simulink model "W03_4_teleop"  (R2024b)
settings: Solver=FixedStepDiscrete  StartTime=0.0  StopTime=T_end_teleop  FixedStep=Ts  RelTol=1e-3
values from neighbouring files (symbols this model uses):
  animate = 1    [W03_setup.m]
  teleop_thrust = 200    [W03_setup.m]
  Ts = 0.05    [W03_setup.m]
libraries: ros2lib x5
settings Model: Creator=admin  LastModifiedBy=admin

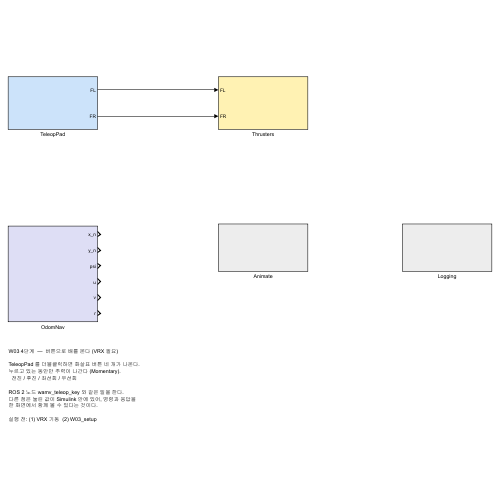
[thumbnail: Simulink's stored preview of the top-level diagram]
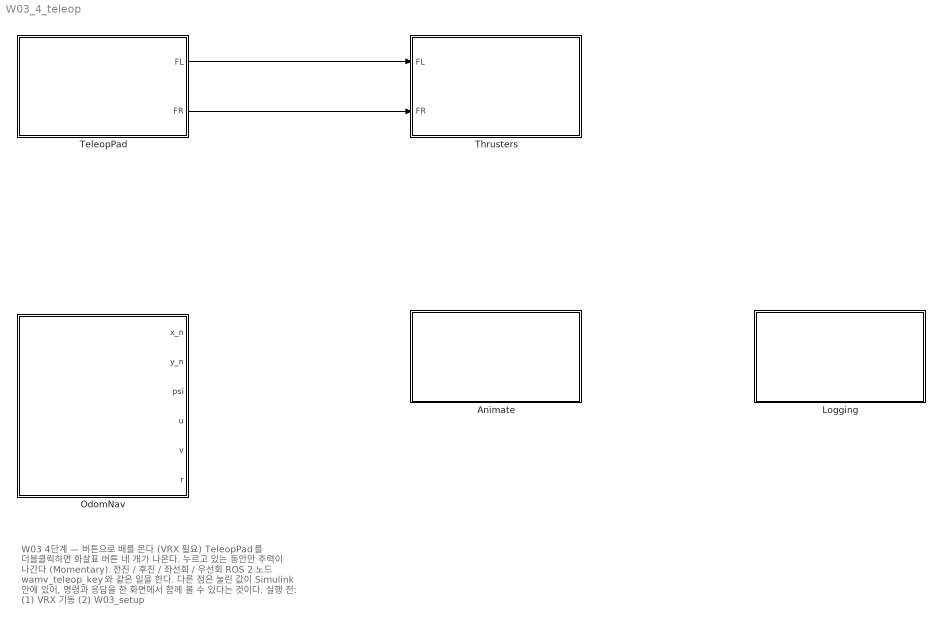
== system W03_4_teleop ==
  note: W03 4단계  —  버튼으로 배를 몬다 (VRX 필요)
      |
      | TeleopPad 를 더블클릭하면 화살표 버튼 네 개가 나온다.
      | 누르고 있는 동안만 추력이 나간다 (Momentary).
      |   전진 / 후진 / 좌선회 / 우선회
      |
      | ROS 2 노드 wamv_teleop_key 와 같은 일을 한다.
      | 다른 점은 눌린 값이 Simulink 안에 있어, 명령과 응답을
      | 한 화면에서 함께 볼 수 있다는 것이다.
      |
      | 실행 전: (1) VRX 기동  (2) W03_setup
  Animate : Subsystem
  Logging : Subsystem
  OdomNav : Subsystem
  TeleopPad : Subsystem
  Thrusters : Subsystem
  wires:
  TeleopPad/1(FL) -> Thrusters/1(FL)
  TeleopPad/2(FR) -> Thrusters/2(FR)

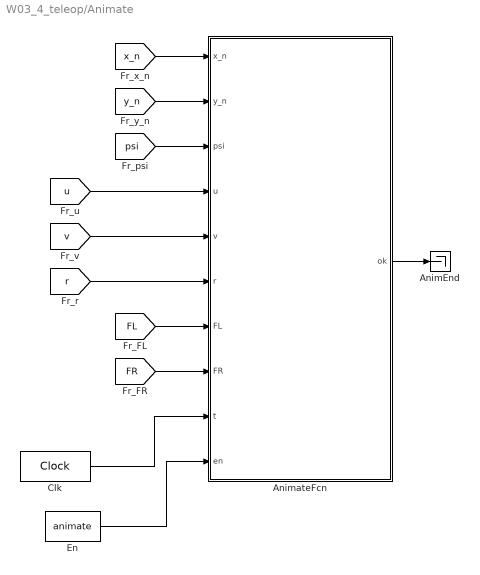
== system W03_4_teleop/Animate ==
  AnimEnd : Terminator
  AnimateFcn : MATLAB Function  TreatAsAtomicUnit=on
  Clk : DigitalClock  SampleTime=Ts
  En : Constant  Value=animate
  wires:
  [r] -> AnimateFcn/6(r)
  [u] -> AnimateFcn/4(u)
  [v] -> AnimateFcn/5(v)
  Clk/1 -> AnimateFcn/9(t)
  En/1 -> AnimateFcn/10(en)
  AnimateFcn/1(ok) -> AnimEnd/1
  [FL] -> AnimateFcn/7(FL)
  [FR] -> AnimateFcn/8(FR)
  [psi] -> AnimateFcn/3(psi)
  [y_n] -> AnimateFcn/2(y_n)
  [x_n] -> AnimateFcn/1(x_n)

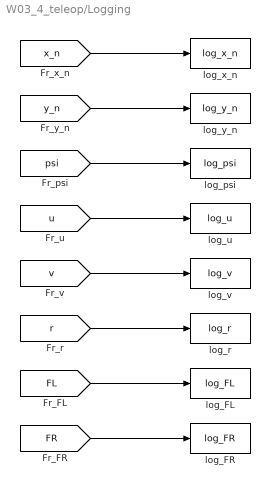
== system W03_4_teleop/Logging ==
  log_FL : ToWorkspace  VariableName=log_FL  SaveFormat=Timeseries  SampleTime=Ts
  log_FR : ToWorkspace  VariableName=log_FR  SaveFormat=Timeseries  SampleTime=Ts
  log_psi : ToWorkspace  VariableName=log_psi  SaveFormat=Timeseries  SampleTime=Ts
  log_r : ToWorkspace  VariableName=log_r  SaveFormat=Timeseries  SampleTime=Ts
  log_u : ToWorkspace  VariableName=log_u  SaveFormat=Timeseries  SampleTime=Ts
  log_v : ToWorkspace  VariableName=log_v  SaveFormat=Timeseries  SampleTime=Ts
  log_x_n : ToWorkspace  VariableName=log_x_n  SaveFormat=Timeseries  SampleTime=Ts
  log_y_n : ToWorkspace  VariableName=log_y_n  SaveFormat=Timeseries  SampleTime=Ts
  wires:
  [x_n] -> log_x_n/1
  [y_n] -> log_y_n/1
  [psi] -> log_psi/1
  [u] -> log_u/1
  [v] -> log_v/1
  [r] -> log_r/1
  [FL] -> log_FL/1
  [FR] -> log_FR/1

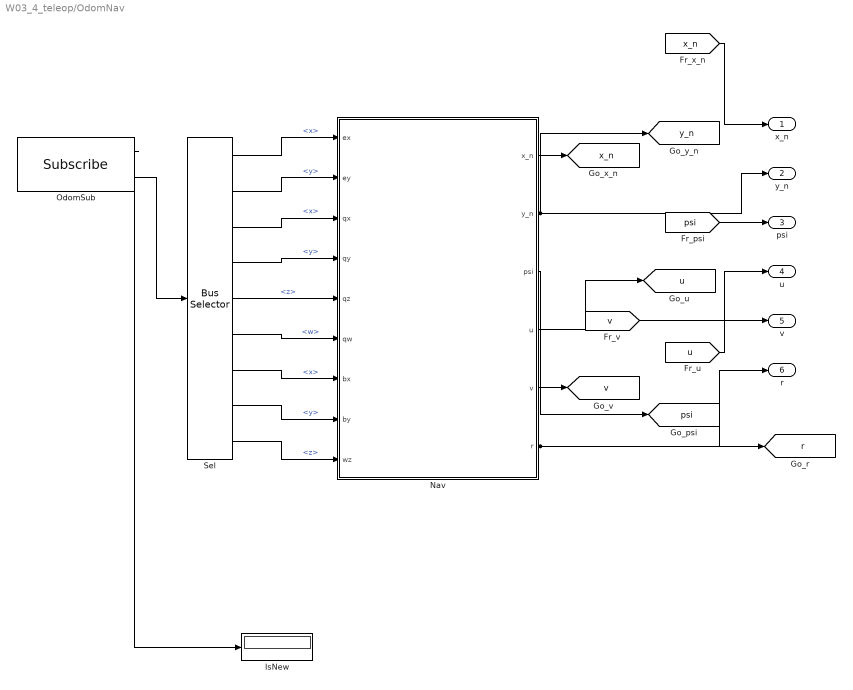
== system W03_4_teleop/OdomNav ==
  IsNew : Display
  Nav : MATLAB Function  TreatAsAtomicUnit=on
  OdomSub : ros2lib/Subscribe  topicSource=Specify your own  topic=/wamv/sensors/position/ground_truth_odometry  messageType=nav_msgs/Odometry  sampleTime=Ts  QOSHistory=Keep last  QOSDepth=1  QOSReliability=Reliable  QOSDurability=Volatile  QOSDeadline=Inf  QOSLifespan=Inf  QOSLiveliness=Automatic  QOSLeaseDuration=Inf  QOSAvoidROSNamespaceConventions=off
  Sel : BusSelector  OutputSignals=pose.pose.position.x,pose.pose.position.y,pose.pose.orientation.x,pose.pose.orientation.y,pose.pose.orientation.z,pose.pose.orientation.w,twist.twist.linear.x,twist.twist.linear.y,twist.twist.angular.z
  x_n : Outport
  y_n : Outport  Port=2
  psi : Outport  Port=3
  u : Outport  Port=4
  v : Outport  Port=5
  r : Outport  Port=6
  tag scope: psi=global, r=global, u=global, v=global, x_n=global, y_n=global
  wires:
  OdomSub/2 -> Sel/1
  Sel/1 -> Nav/1(ex)  "<x>"
  Sel/2 -> Nav/2(ey)  "<y>"
  Sel/3 -> Nav/3(qx)  "<x>"
  Sel/4 -> Nav/4(qy)  "<y>"
  Sel/5 -> Nav/5(qz)  "<z>"
  Sel/6 -> Nav/6(qw)  "<w>"
  Sel/7 -> Nav/7(bx)  "<x>"
  Sel/8 -> Nav/8(by)  "<y>"
  Sel/9 -> Nav/9(wz)  "<z>"
  Nav/2(y_n) -> y_n/1, [y_n]
  Nav/4(u) -> [u]
  OdomSub/1 -> IsNew/1
  Nav/5(v) -> [v]
  Nav/1(x_n) -> [x_n]
  [psi] -> psi/1
  [v] -> v/1
  Nav/6(r) -> [r], r/1
  Nav/3(psi) -> [psi]
  [u] -> u/1
  [x_n] -> x_n/1

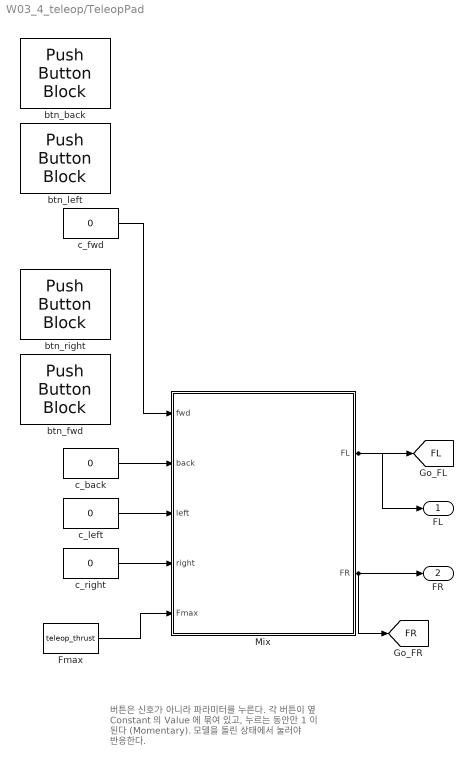
== system W03_4_teleop/TeleopPad ==
  note: 버튼은 신호가 아니라 파라미터를 누른다.
      | 각 버튼이 옆 Constant 의 Value 에 묶여 있고,
      | 누르는 동안만 1 이 된다 (Momentary).
      | 모델을 돌린 상태에서 눌러야 반응한다.
  Fmax : Constant  Value=teleop_thrust
  Mix : MATLAB Function  TreatAsAtomicUnit=on
  btn_back : PushButtonBlock  ButtonText=▼ 후진
  btn_fwd : PushButtonBlock  ButtonText=▲ 전진
  btn_left : PushButtonBlock  ButtonText=◀ 좌선회
  btn_right : PushButtonBlock  ButtonText=▶ 우선회
  c_back : Constant  Value=0
  c_fwd : Constant  Value=0
  c_left : Constant  Value=0
  c_right : Constant  Value=0
  FL : Outport
  FR : Outport  Port=2
  tag scope: FL=global, FR=global
  wires:
  c_left/1 -> Mix/3(left)
  c_fwd/1 -> Mix/1(fwd)
  c_back/1 -> Mix/2(back)
  c_right/1 -> Mix/4(right)
  Fmax/1 -> Mix/5(Fmax)
  Mix/1(FL) -> FL/1, [FL]
  Mix/2(FR) -> FR/1, [FR]

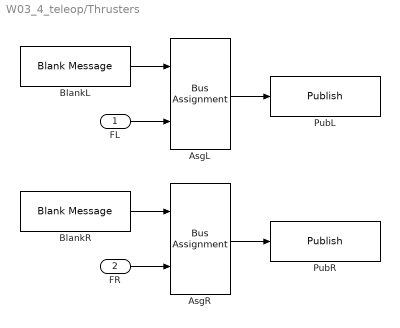
== system W03_4_teleop/Thrusters ==
  FL : Inport
  FR : Inport  Port=2
  AsgL : BusAssignment  AssignedSignals=data
  AsgR : BusAssignment  AssignedSignals=data
  BlankL : ros2lib/Blank Message  messageClass=Message  entityType=std_msgs/Float64  messageType=std_msgs/Float64  SampleTime=Ts
  BlankR : ros2lib/Blank Message  messageClass=Message  entityType=std_msgs/Float64  messageType=std_msgs/Float64  SampleTime=Ts
  PubL : ros2lib/Publish  topicSource=Specify your own  topic=/wamv/thrusters/left/thrust  messageType=std_msgs/Float64  QOSHistory=Keep last  QOSDepth=1  QOSReliability=Reliable  QOSDurability=Volatile  QOSDeadline=Inf  QOSLifespan=Inf  QOSLiveliness=Automatic  QOSLeaseDuration=Inf  QOSAvoidROSNamespaceConventions=off
  PubR : ros2lib/Publish  topicSource=Specify your own  topic=/wamv/thrusters/right/thrust  messageType=std_msgs/Float64  QOSHistory=Keep last  QOSDepth=1  QOSReliability=Reliable  QOSDurability=Volatile  QOSDeadline=Inf  QOSLifespan=Inf  QOSLiveliness=Automatic  QOSLeaseDuration=Inf  QOSAvoidROSNamespaceConventions=off
  wires:
  AsgR/1 -> PubR/1
  BlankL/1 -> AsgL/1
  FL/1 -> AsgL/2
  BlankR/1 -> AsgR/1
  FR/1 -> AsgR/2
  AsgL/1 -> PubL/1

== matlab function W03_4_teleop/OdomNav/Nav ==
  data: ex input; x_n output; ey input; qx input; qy input; qz input; qw input; bx input; by input; wz input; y_n output; psi output; u output; v output; r output
function [x_n, y_n, psi, u, v, r] = Nav(ex, ey, qx, qy, qz, qw, bx, by, wz)
%#codegen
% odometry 하나로 위치·자세·속도를 모두 얻는다 (ENU -> NED).
%   위치   x_n = ey,  y_n = ex      ENU 의 y 가 북, x 가 동
%   자세   psi = pi/2 - yaw_ENU
%   속도   u = bx,  v = -by,  r = -wz   y·z 축이 뒤집히므로 부호가 바뀐다
%
% 기준점은 첫 메시지의 위치로 잡는다. 그래야 항적이 (0,0) 에서 시작한다.
persistent x0 y0 seen
if isempty(seen), seen = false; x0 = 0; y0 = 0; end

xr = ey;   yr = ex;
if ~seen && (abs(ex) + abs(ey)) > 0
    seen = true;  x0 = xr;  y0 = yr;
end
x_n = xr - x0;
y_n = yr - y0;

yaw_enu = atan2(2*(qw*qz + qx*qy), 1 - 2*(qy*qy + qz*qz));
p   = pi/2 - yaw_enu;
psi = atan2(sin(p), cos(p));

u =  bx;
v = -by;
r = -wz;

== matlab function W03_4_teleop/TeleopPad/Mix ==
  data: fwd input; FL output; back input; left input; right input; Fmax input; FR output
function [FL, FR] = Mix(fwd, back, left, right, Fmax)
%#codegen
% wamv_teleop_key 와 같은 차동 배분.
%   전진   FL = +F, FR = +F      후진   FL = -F, FR = -F
%   좌선회 FL = -F, FR = +F      우선회 FL = +F, FR = -F
%
% 좌선회에서 요 모멘트 N = (FL - FR)*b 가 음수라 psi_NED 가 줄어든다.
surge = fwd   - back;
turn  = right - left;
FL = Fmax*(surge + turn);
FR = Fmax*(surge - turn);
FL = min(max(FL, -Fmax), Fmax);
FR = min(max(FR, -Fmax), Fmax);

== matlab function W03_4_teleop/Animate/AnimateFcn ==
  data: x_n input; y_n input; psi input; u input; ok output; v input; r input; FL input; FR input; t input; en input
function ok = AnimateFcn(x_n, y_n, psi, u, v, r, FL, FR, t, en)
%#codegen
% 그림은 코드 생성 대상이 아니므로 extrinsic 으로 부른다.
coder.extrinsic('W03_teleop_plot');
ok = 1;
if en > 0.5
    W03_teleop_plot(x_n, y_n, psi, u, v, r, FL, FR, t);
end
